simulink model "modelo_SIR"  (R2019b)
settings: Solver=VariableStepAuto  StartTime=0.0  StopTime=365  RelTol=1e-3
settings Model: Creator=lucia  LastModifiedBy=lucia

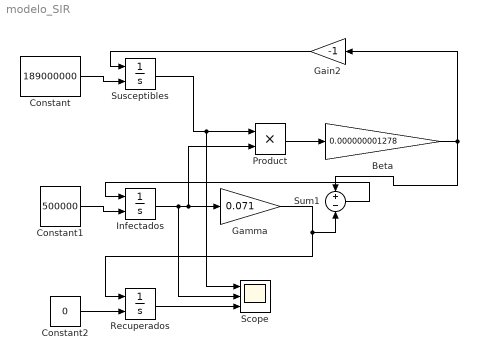
== system modelo_SIR ==
  Beta : Gain  Gain=0.000000001278
  Constant : Constant  Value=189000000
  Constant1 : Constant  Value=500000
  Constant2 : Constant  Value=0
  Gain2 : Gain  Gain=-1
  Gamma : Gain  Gain=0.071
  Infectados : Integrator  InitialConditionSource=external
  Product : Product
  Recuperados : Integrator  InitialConditionSource=external
  Scope : Scope  NumInputPorts=3
  Sum1 : Sum  Inputs=+-
  Susceptibles : Integrator  InitialConditionSource=external
  wires:
  Constant/1 -> Susceptibles/2
  Constant1/1 -> Infectados/2
  Constant2/1 -> Recuperados/2
  Susceptibles/1 -> Scope/1, Product/1
  Infectados/1 -> Scope/2, Product/2, Gamma/1
  Product/1 -> Beta/1
  Beta/1 -> Gain2/1, Sum1/1
  Sum1/1 -> Infectados/1
  Recuperados/1 -> Scope/3
  Gamma/1 -> Recuperados/1, Sum1/2
  Gain2/1 -> Susceptibles/1
